simulink model "Drone_2M_sim_V8_OnlyForReport"  (R2022a)
settings: Solver=VariableStepAuto  StartTime=0.0  StopTime=SIM_TIME  RelTol=1e-3
undefined symbols (not defined in the file): batteryMass, batteryPositionOffset, batVolt, body, bodyMass, calibServo, deadCurrent, denumRollYawFF, disableWallSensor, Dist, enableRollToYaw, footZ, h1al, h1iuse, h1kp, h1td, h1ti, hoverControl, hoverVoltage, hval, hviuse, hvkp, hvtd, hvti, KDrag, Km, Ktrust, leftDeadBandWidthDeg, minimumMotorVolt, motorMass, noiseOn, numRollYawFF, paal, pakp, patd, pati, patiuse, pitch_act_lim, pitchCalibGain, pitchStepSize, pitchVelIntLimit, propellerMass, pval, pvkp, pvtd, pvti, pvtiuse, Ra, raal, radToDeg, rakp, ral, ratd, rati, ratiuse, rightDeadBandWidthDeg, rkp, roll_act_lim, roll_limit, rollCalibGain ... (+72)
libraries: sm_lib x86, nesl_utility x40, sharedtransform x1
(part 4 of 4)

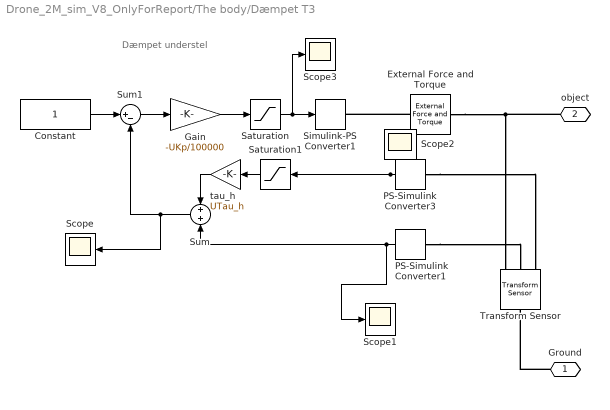
== system Drone_2M_sim_V8_OnlyForReport/The body/Dæmpet T3 ==
  note: Dæmpet understel
  Constant : Constant
  External Force and Torque : sm_lib/Forces and Torques/External Force and Torque  ForceResolutionFrame=AttachedFrame  EnableForceX=on  EnableForceY=off  EnableForceZ=off  EnableForce=off  TorqueResolutionFrame=AttachedFrame  EnableTorqueX=off  EnableTorqueY=off  EnableTorqueZ=off  EnableTorque=off
  Gain : Gain  Gain=-UKp/100000
  PS-Simulink Converter1 : nesl_utility/PS-Simulink Converter  PhysicalDomain=network_engine_domain  SubClassName=ps_output  LeftPortType=input  RightPortType=output  PseudoPeriodic=off  Frequencies=[]  VectorFormat=1-D array  Unit=1  AffineConversion=off
      settings: SourceProductBaseCode=SS,PW,VE
  PS-Simulink Converter3 : nesl_utility/PS-Simulink Converter  PhysicalDomain=network_engine_domain  SubClassName=ps_output  LeftPortType=input  RightPortType=output  PseudoPeriodic=off  Frequencies=[]  VectorFormat=1-D array  Unit=1  AffineConversion=off
      settings: SourceProductBaseCode=SS,PW,VE
  Saturation : Saturate  UpperLimit=ULimit/100000  LowerLimit=0
  Saturation1 : Saturate  UpperLimit=0.2  LowerLimit=-0.2
  Scope{,1..3} (4 alike) : Scope
  Simulink-PS Converter1 : nesl_utility/Simulink-PS Converter  PhysicalDomain=network_engine_domain  SubClassName=ps_input  LeftPortType=input  RightPortType=output  PseudoPeriodic=off  Frequencies=[]  NoiseDistribution=none  NoiseParameters=[]  Unit=1  AffineConversion=off  FilteringAndDerivatives=zero  SimscapeFilterOrder=1  InputFilterTimeConstant=0.001  UdotUserProvided=1
      settings: SourceProductBaseCode=SS,PW,VE
  Sum : Sum  Inputs=+|+
  Sum1 : Sum  Inputs=|+-
  Transform Sensor : sm_lib/Frames and Transforms/Transform Sensor  MeasurementFrame=World  SenseAngle=off  SenseAxis=off  SenseAngle1=off  SenseAngle2=off  SenseAngle3=off  SenseQ=off  SenseR=off  SenseOmegaX=off  SenseOmegaY=off  SenseOmegaZ=off  SenseOmega1=off  SenseOmega2=off  SenseOmega3=off  SenseQDot=off  SenseRDot=off  SenseAlphaX=off  SenseAlphaY=off  SenseAlphaZ=off  SenseAlpha1=off  SenseAlpha2=off  SenseAlpha3=off  SenseQDDot=off  SenseRDDot=off  SenseX=on  SenseY=off  SenseZ=off  SenseRad=off  SenseAzim=off  SenseDist=off  SenseInc=off  SenseXDot=on  SenseYDot=off  SenseZDot=off  SenseRadDot=off  SenseAzimDot=off  SenseDistDot=off  SenseIncDot=off  SenseXDDot=off  SenseYDDot=off  SenseZDDot=off  SenseRadDDot=off  SenseAzimDDot=off  SenseDistDDot=off  SenseIncDDot=off
  tau_h : Gain  Gain=UTau_h
  Ground : PMIOPort  Side=Left
  object : PMIOPort  Port=2  Side=Right
  wires:
  Constant/1 -> Sum1/1
  Sum1/1 -> Gain/1
  Saturation/1 -> Scope3/1, Simulink-PS Converter1/1
  Gain/1 -> Saturation/1
  Saturation1/1 -> tau_h/1
  tau_h/1 -> Sum/1
  Sum/1 -> Scope/1, Sum1/2
  PS-Simulink Converter3/1 -> Saturation1/1, Scope2/1
  PS-Simulink Converter1/1 -> Sum/2, Scope1/1
  connections:
  PS-Simulink Converter3/LConn1 -- Transform Sensor/RConn3
  PS-Simulink Converter1/LConn1 -- Transform Sensor/RConn2
  External Force and Torque/LConn1 -- Simulink-PS Converter1/RConn1
  External Force and Torque/RConn1 -- Transform Sensor/RConn1 -- object/RConn1
  Ground/RConn1 -- Transform Sensor/LConn1

== system Drone_2M_sim_V8_OnlyForReport/The body/Dæmpet til gulvet ==
  note: Dæmpet understel
  Constant : Constant  Value=0
  External Force and Torque : sm_lib/Forces and Torques/External Force and Torque  ForceResolutionFrame=AttachedFrame  EnableForceX=off  EnableForceY=off  EnableForceZ=on  EnableForce=off  TorqueResolutionFrame=AttachedFrame  EnableTorqueX=off  EnableTorqueY=off  EnableTorqueZ=off  EnableTorque=off
  Gain : Gain  Gain=UKp
  PS-Simulink Converter1 : nesl_utility/PS-Simulink Converter  PhysicalDomain=network_engine_domain  SubClassName=ps_output  LeftPortType=input  RightPortType=output  PseudoPeriodic=off  Frequencies=[]  VectorFormat=1-D array  Unit=1  AffineConversion=off
      settings: SourceProductBaseCode=SS,PW,VE
  PS-Simulink Converter3 : nesl_utility/PS-Simulink Converter  PhysicalDomain=network_engine_domain  SubClassName=ps_output  LeftPortType=input  RightPortType=output  PseudoPeriodic=off  Frequencies=[]  VectorFormat=1-D array  Unit=1  AffineConversion=off
      settings: SourceProductBaseCode=SS,PW,VE
  Saturation : Saturate  UpperLimit=ULimit  LowerLimit=0
  Saturation1 : Saturate  UpperLimit=0.2  LowerLimit=-0.2
  Scope{,1..3} (4 alike) : Scope
  Simulink-PS Converter1 : nesl_utility/Simulink-PS Converter  PhysicalDomain=network_engine_domain  SubClassName=ps_input  LeftPortType=input  RightPortType=output  PseudoPeriodic=off  Frequencies=[]  NoiseDistribution=none  NoiseParameters=[]  Unit=1  AffineConversion=off  FilteringAndDerivatives=zero  SimscapeFilterOrder=1  InputFilterTimeConstant=0.001  UdotUserProvided=1
      settings: SourceProductBaseCode=SS,PW,VE
  Sum : Sum  Inputs=+|+
  Sum1 : Sum  Inputs=|+-
  Transform Sensor : sm_lib/Frames and Transforms/Transform Sensor  MeasurementFrame=World  SenseAngle=off  SenseAxis=off  SenseAngle1=off  SenseAngle2=off  SenseAngle3=off  SenseQ=off  SenseR=off  SenseOmegaX=off  SenseOmegaY=off  SenseOmegaZ=off  SenseOmega1=off  SenseOmega2=off  SenseOmega3=off  SenseQDot=off  SenseRDot=off  SenseAlphaX=off  SenseAlphaY=off  SenseAlphaZ=off  SenseAlpha1=off  SenseAlpha2=off  SenseAlpha3=off  SenseQDDot=off  SenseRDDot=off  SenseX=off  SenseY=off  SenseZ=on  SenseRad=off  SenseAzim=off  SenseDist=off  SenseInc=off  SenseXDot=off  SenseYDot=off  SenseZDot=on  SenseRadDot=off  SenseAzimDot=off  SenseDistDot=off  SenseIncDot=off  SenseXDDot=off  SenseYDDot=off  SenseZDDot=off  SenseRadDDot=off  SenseAzimDDot=off  SenseDistDDot=off  SenseIncDDot=off
  tau_h : Gain  Gain=UTau_h
  Ground : PMIOPort  Side=Left
  object : PMIOPort  Port=2  Side=Right
  wires:
  Constant/1 -> Sum1/1
  Sum1/1 -> Gain/1
  Saturation/1 -> Scope3/1, Simulink-PS Converter1/1
  Gain/1 -> Saturation/1
  Saturation1/1 -> tau_h/1
  tau_h/1 -> Sum/1
  Sum/1 -> Scope/1, Sum1/2
  PS-Simulink Converter3/1 -> Saturation1/1, Scope2/1
  PS-Simulink Converter1/1 -> Sum/2, Scope1/1
  connections:
  PS-Simulink Converter3/LConn1 -- Transform Sensor/RConn3
  PS-Simulink Converter1/LConn1 -- Transform Sensor/RConn2
  External Force and Torque/LConn1 -- Simulink-PS Converter1/RConn1
  External Force and Torque/RConn1 -- Transform Sensor/RConn1 -- object/RConn1
  Ground/RConn1 -- Transform Sensor/LConn1

== system Drone_2M_sim_V8_OnlyForReport/Control units/height_control/height ctrl1 ==
  ref : Inport
  measurement : Inport  Port=2
  Constant : Constant  Value=0
  Gain : Gain  Gain=h1kp
  Gain1 : Gain  Gain=h1iuse/h1ti
  Integrator : Integrator  InitialConditionSource=external  InitialCondition=minimumMotorVolt  LimitOutput=on  UpperSaturationLimit=10  LowerSaturationLimit=-10
  Mux1 : Mux  Inputs=3
  Mux3 : Mux
  Sum : Sum  Inputs=|+-
  Sum1 : Sum  Inputs=|++
  Transfer Fcn : TransferFcn  Numerator=[h1td 1]  Denominator=[h1al*h1td 1]
  height-control-in : Scope
  height-control-out : Scope
  u : Outport  VectorParamsAs1DForOutWhenUnconnected=off
  wires:
  Transfer Fcn/1 -> Sum/2, Mux3/3  "m2"
  Mux1/1 -> height-control-out/1
  Gain/1 -> Gain1/1, Mux1/2, Sum1/2  "eKp"
  Sum1/1 -> u/1, Mux1/3  "u"
  Mux3/1 -> height-control-in/1
  Gain1/1 -> Integrator/1
  Integrator/1 -> Sum1/1, Mux1/1  "i"
  Sum/1 -> Gain/1, Mux3/1  "e"
  measurement/1 -> Transfer Fcn/1, Mux3/2  "m1"
  ref/1 -> Sum/1, Mux3/4  "ref"
  Constant/1 -> Integrator/2

== system Drone_2M_sim_V8_OnlyForReport/Control units/height_control/height vel ctrl ==
  ref : Inport
  measurement : Inport  Port=2
  Constant : Constant  Value=hoverControl
  Gain : Gain  Gain=hvkp
  Gain1 : Gain  Gain=hviuse/hvti
  Integrator : Integrator  InitialConditionSource=external  InitialCondition=minimumMotorVolt  LimitOutput=on  UpperSaturationLimit=1000  LowerSaturationLimit=-1000
  Mux1 : Mux  Inputs=3
  Mux3 : Mux
  Saturation6 : Saturate  UpperLimit=trust_lim  LowerLimit=0
  Sum : Sum  Inputs=|+-
  Sum1 : Sum  Inputs=|++
  Transfer Fcn : TransferFcn  Numerator=[hvtd 1]  Denominator=[hval*hvtd 1]
  height-control-in : Scope
  height-control-out : Scope
  u : Outport  VectorParamsAs1DForOutWhenUnconnected=off
  wires:
  ref/1 -> Mux3/4, Sum/1  "ref"
  measurement/1 -> Mux3/2, Transfer Fcn/1  "m1"
  Sum/1 -> Mux3/1, Gain/1  "e"
  Integrator/1 -> Sum1/1, Mux1/1  "i"
  Gain1/1 -> Integrator/1
  Mux3/1 -> height-control-in/1
  Saturation6/1 -> Mux1/3, u/1  "u"
  Gain/1 -> Sum1/2, Mux1/2, Gain1/1  "eKp"
  Mux1/1 -> height-control-out/1
  Sum1/1 -> Saturation6/1
  Transfer Fcn/1 -> Mux3/3, Sum/2  "m2"
  Constant/1 -> Integrator/2

== system Drone_2M_sim_V8_OnlyForReport/Control units/yaw ctrl/angle_lin_pm_pi ==
  rad-in : Inport
  Atan2 : Trigonometry  Operator=atan2
  Sin : Trigonometry
  Sin1 : Trigonometry  Operator=cos
  rad-out : Outport
  wires:
  Atan2/1 -> rad-out/1
  Sin/1 -> Atan2/1
  rad-in/1 -> Sin/1, Sin1/1
  Sin1/1 -> Atan2/2

== system Drone_2M_sim_V8_OnlyForReport/Motors/Servo_left/Signal Builder ==
  Demux : Demux  Tag=STV Demux  Outputs=1
      settings: DisplayOption=none
  FromWs : FromWorkspace  Tag=STV FromWs  VariableName=tuvar
      SigBuilderData=|
      | common.afterFinalStr = 'Extrapolate'
      | common.sampleTime = 0
      | dataSet.timeRange = [0 30]
      | dataSet.name = 'Group 1'
      | sbobj.Groups.Name = 'Group 1'
      | sbobj.Groups.Signals.Name = 'Signal 1'
      | sbobj.Groups.Signals.XData = [0 4.5 4.5 10 10 30]
      | sbobj.Groups.Signals.YData = [0 0 1 1 0 0]
      | sbobj.Groups.TimeRange = [0 30]
  Signal 1 : Outport  Tag=STV Outport
  wires:
  Demux/1 -> Signal 1/1
  FromWs/1 -> Demux/1

== system Drone_2M_sim_V8_OnlyForReport/Motors/Servo_left/Signal Builder1 ==
  Demux : Demux  Tag=STV Demux  Outputs=1
      settings: DisplayOption=none
  FromWs : FromWorkspace  Tag=STV FromWs  VariableName=tuvar
      SigBuilderData=|
      | common.afterFinalStr = 'Extrapolate'
      | common.sampleTime = 0
      | dataSet.timeRange = [0 30]
      | dataSet.name = 'Group 1'
      | sbobj.Groups.Name = 'Group 1'
      | sbobj.Groups.Signals.Name = 'Signal 1'
      | sbobj.Groups.Signals.XData = [0 4 4 10 10 30]
      | sbobj.Groups.Signals.YData = [0 0 1 1 0 0]
      | sbobj.Groups.TimeRange = [0 30]
  Signal 1 : Outport  Tag=STV Outport
  wires:
  Demux/1 -> Signal 1/1
  FromWs/1 -> Demux/1

== system Drone_2M_sim_V8_OnlyForReport/Motors/Servo_right/Signal Builder ==
  Demux : Demux  Tag=STV Demux  Outputs=1
      settings: DisplayOption=none
  FromWs : FromWorkspace  Tag=STV FromWs  VariableName=tuvar
      SigBuilderData=|
      | common.afterFinalStr = 'Extrapolate'
      | common.sampleTime = 0
      | dataSet.timeRange = [0 30]
      | dataSet.name = 'Group 1'
      | sbobj.Groups.Name = 'Group 1'
      | sbobj.Groups.Signals.Name = 'Signal 1'
      | sbobj.Groups.Signals.XData = [0 4.5 4.5 10 10 30]
      | sbobj.Groups.Signals.YData = [0 0 1 1 0 0]
      | sbobj.Groups.TimeRange = [0 30]
  Signal 1 : Outport  Tag=STV Outport
  wires:
  Demux/1 -> Signal 1/1
  FromWs/1 -> Demux/1

== system Drone_2M_sim_V8_OnlyForReport/Motors/Servo_right/Signal Builder1 ==
  Demux : Demux  Tag=STV Demux  Outputs=1
      settings: DisplayOption=none
  FromWs : FromWorkspace  Tag=STV FromWs  VariableName=tuvar
      SigBuilderData=|
      | common.afterFinalStr = 'Extrapolate'
      | common.sampleTime = 0
      | dataSet.timeRange = [0 30]
      | dataSet.name = 'Group 1'
      | sbobj.Groups.Name = 'Group 1'
      | sbobj.Groups.Signals.Name = 'Signal 1'
      | sbobj.Groups.Signals.XData = [0 4 4 10 10 30]
      | sbobj.Groups.Signals.YData = [0 0 1 1 0 0]
      | sbobj.Groups.TimeRange = [0 30]
  Signal 1 : Outport  Tag=STV Outport
  wires:
  Demux/1 -> Signal 1/1
  FromWs/1 -> Demux/1
